simulink model "quadcopter_rl_env"  (R2024b)
settings: Solver=ode4  StartTime=0.0  StopTime=T_episode  FixedStep=Ts_inner  RelTol=1e-3
undefined symbols (not defined in the file): alpha, Kd_phi, Kd_psi, Kd_theta, Kd_x, Kd_y, Kd_z, Ki_phi, Ki_psi, Ki_theta, Ki_x, Ki_y, Ki_z, Kp_phi, Kp_psi, Kp_theta, Kp_x, Kp_y, Kp_z, psi_d, wind_force_N, wind_onset_time, x_d, y_d, z_d
libraries: slpidlib x6, rllib x1
settings Model: Creator=hridd  LastModifiedBy=hridd

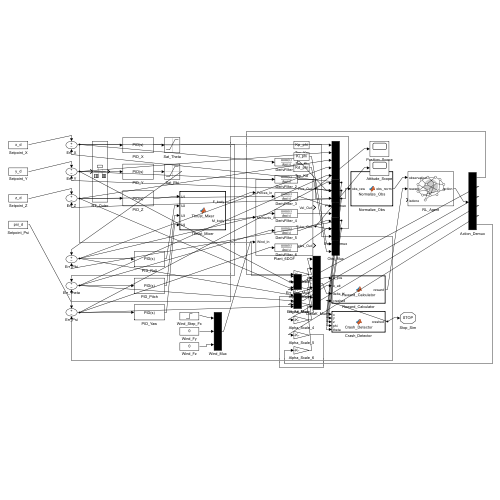
[thumbnail: Simulink's stored preview of the top-level diagram]
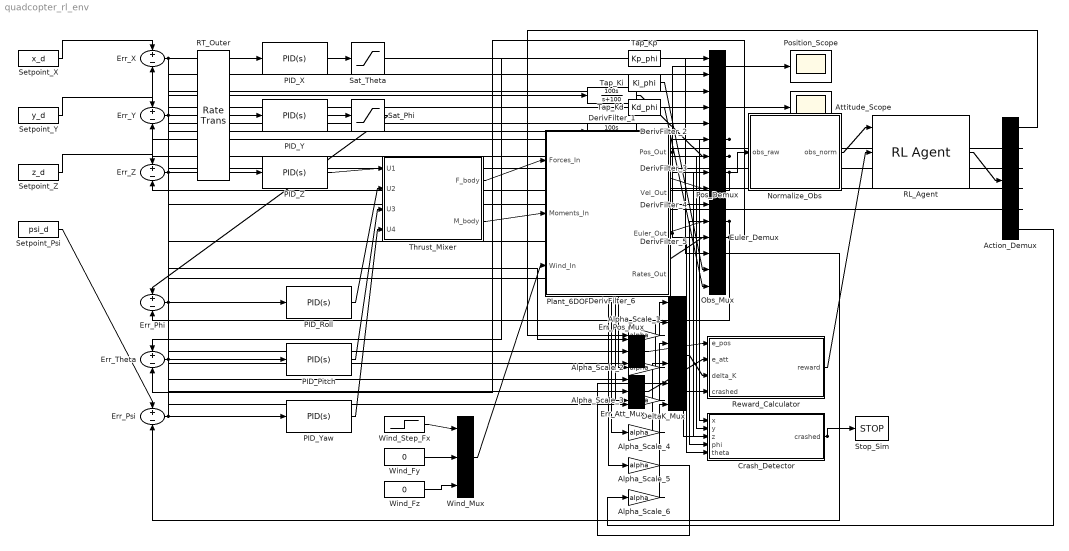
== system quadcopter_rl_env ==
  Action_Demux : Demux  Outputs=6
  Alpha_Scale_{1..6} (6 alike) : Gain  Gain=alpha
  Attitude_Scope : Scope
  Crash_Detector : MATLAB Function  TreatAsAtomicUnit=on
  DeltaK_Mux : Mux  Inputs=6
  DerivFilter_{1..6} (6 alike) : TransferFcn  Numerator=[100 0]  Denominator=[1 100]
  Err_Att_Mux : Mux  Inputs=3
  Err_Phi : Sum  Inputs=+-
  Err_Pos_Mux : Mux  Inputs=3
  Err_Psi : Sum  Inputs=+-
  Err_Theta : Sum  Inputs=+-
  Err_X : Sum  Inputs=+-
  Err_Y : Sum  Inputs=+-
  Err_Z : Sum  Inputs=+-
  Euler_Demux : Demux  Outputs=3
  Normalize_Obs : MATLAB Function  TreatAsAtomicUnit=on
  Obs_Mux : Mux  Inputs=15
  PID_Pitch : slpidlib/PID Controller  Controller=PID  Form=Parallel  TimeDomain=Continuous-time  UseExternalTs=off  SampleTime=-1  IntegratorMethod=Forward Euler  FilterMethod=Forward Euler  ControllerParametersSource=internal  P=Kp_theta  I=Ki_theta  UseKiTs=off  D=Kd_theta  UseExternalDerivativeSource=off  N=100  UseFilter=on  TunerSelectOption=Transfer Function Based (PID Tuner App)  InitialConditionSource=internal  InitialConditionForIntegrator=0  InitialConditionForFilter=0  DifferentiatorICPrevScaledInput=0  ExternalReset=none  TrackingMode=off  Kt=1  LimitOutput=off  SatLimitsSource=internal  UpperSaturationLimit=inf  LowerSaturationLimit=-inf  LinearizeAsGain=on  AntiWindupMode=none  Kb=1  LimitIntegrator=off  UpperIntegratorSaturationLimit=inf  LowerIntegratorSaturationLimit=-inf  POutMin=[]  POutMax=[]  IOutMin=[]  IOutMax=[]  DOutMin=[]  DOutMax=[]  NOutMin=[]  NOutMax=[]  SumOutMin=[]  SumOutMax=[]  SaturationOutMin=[]  SaturationOutMax=[]  PParamMin=[]  PParamMax=[]  IParamMin=[]  IParamMax=[]  DParamMin=[]  DParamMax=[]  NParamMin=[]  NParamMax=[]  KbParamMin=[]  KbParamMax=[]  KtParamMin=[]  KtParamMax=[]  KbOutMin=[]  KbOutMax=[]  KtOutMin=[]  KtOutMax=[]  IntegratorOutMin=[]  IntegratorOutMax=[]  FilterOutMin=[]  FilterOutMax=[]  SumI1OutMin=[]  SumI1OutMax=[]  SumI2OutMin=[]  SumI2OutMax=[]  SumI3OutMin=[]  SumI3OutMax=[]  SumI4OutMin=[]  SumI4OutMax=[]  SumDOutMin=[]  SumDOutMax=[]  DifferentiatorOutMin=[]  DifferentiatorOutMax=[]  FilterDiffOutCoefMin=[]  FilterDiffOutCoefMax=[]  ReciprocalOutMin=[]  ReciprocalOutMax=[]  SumDenOutMin=[]  SumDenOutMax=[]  SumNumOutMin=[]  SumNumOutMax=[]  DivideOutMin=[]  DivideOutMax=[]  UdiffTsProdOutMin=[]  UdiffTsProdOutMax=[]  NTsProdOutMin=[]  NTsProdOutMax=[]  UintegralTsProdOutMin=[]  UintegralTsProdOutMax=[]  UngainTsProdOutMin=[]  UngainTsProdOutMax=[]  ClampingZeroOutDataTypeStr=Inherit: Inherit via back propagation  ClampingZeroOutMin=[]  ClampingZeroOutMax=[]  FilterDenConstantOutDataTypeStr=Inherit: Inherit via back propagation  FilterDenConstantOutMin=[]  FilterDenConstantOutMax=[]  PCopyOutDataTypeStr=Inherit: Inherit via back propagation  PCopyOutMin=[]  PCopyOutMax=[]  NCopyOutDataTypeStr=Inherit: Inherit via back propagation  NCopyOutMin=[]  NCopyOutMax=[]  IntegratorContinuousStateAttributes=''  IntegratorStateMustResolveToSignalObject=off  IntegratorRTWStateStorageClass=Auto  FilterContinuousStateAttributes=''  FilterStateMustResolveToSignalObject=off  FilterRTWStateStorageClass=Auto  ParallelPVariant=InternalParameters  IdealPVariant=Disabled  IVariant=InternalParameters  DVariant=InternalParameters  IntegratorVariant=Continuous  SatVariant=Disabled  AWVariant=Passthrough  PCopyVariant=Disabled  TRVariant=Disabled  FdbkBlocksVariant=Forward  IdealPFdbkVariant=Disabled  SatFdbkVariant=Disabled  DerivativeFilterVariant=ContFilter  NVariant=InternalParameters  NCopyVariant=Disabled  FilterICVariant=InternalICsFilter  IntegratorICVariant=InternalICs  ExternalResetVariant=Disabled  TRSumVariant=Passthrough  SumFdbkVariant=Disabled  SumVariant=Sum_PID  TsampFilterVariant=InternalTs  TsampNgainVariant=Passthrough  TsampIntegralVariant=Disabled_SignalSpec  ExternalSaturationOutDataTypeStr=Inherit: Same as second input  DerivativeSourceVariant=ErrorSignal  PreIntVariant=InternalPreInt
  PID_Roll : slpidlib/PID Controller  Controller=PID  Form=Parallel  TimeDomain=Continuous-time  UseExternalTs=off  SampleTime=-1  IntegratorMethod=Forward Euler  FilterMethod=Forward Euler  ControllerParametersSource=internal  P=Kp_phi  I=Ki_phi  UseKiTs=off  D=Kd_phi  UseExternalDerivativeSource=off  N=100  UseFilter=on  TunerSelectOption=Transfer Function Based (PID Tuner App)  InitialConditionSource=internal  InitialConditionForIntegrator=0  InitialConditionForFilter=0  DifferentiatorICPrevScaledInput=0  ExternalReset=none  TrackingMode=off  Kt=1  LimitOutput=off  SatLimitsSource=internal  UpperSaturationLimit=inf  LowerSaturationLimit=-inf  LinearizeAsGain=on  AntiWindupMode=none  Kb=1  LimitIntegrator=off  UpperIntegratorSaturationLimit=inf  LowerIntegratorSaturationLimit=-inf  POutMin=[]  POutMax=[]  IOutMin=[]  IOutMax=[]  DOutMin=[]  DOutMax=[]  NOutMin=[]  NOutMax=[]  SumOutMin=[]  SumOutMax=[]  SaturationOutMin=[]  SaturationOutMax=[]  PParamMin=[]  PParamMax=[]  IParamMin=[]  IParamMax=[]  DParamMin=[]  DParamMax=[]  NParamMin=[]  NParamMax=[]  KbParamMin=[]  KbParamMax=[]  KtParamMin=[]  KtParamMax=[]  KbOutMin=[]  KbOutMax=[]  KtOutMin=[]  KtOutMax=[]  IntegratorOutMin=[]  IntegratorOutMax=[]  FilterOutMin=[]  FilterOutMax=[]  SumI1OutMin=[]  SumI1OutMax=[]  SumI2OutMin=[]  SumI2OutMax=[]  SumI3OutMin=[]  SumI3OutMax=[]  SumI4OutMin=[]  SumI4OutMax=[]  SumDOutMin=[]  SumDOutMax=[]  DifferentiatorOutMin=[]  DifferentiatorOutMax=[]  FilterDiffOutCoefMin=[]  FilterDiffOutCoefMax=[]  ReciprocalOutMin=[]  ReciprocalOutMax=[]  SumDenOutMin=[]  SumDenOutMax=[]  SumNumOutMin=[]  SumNumOutMax=[]  DivideOutMin=[]  DivideOutMax=[]  UdiffTsProdOutMin=[]  UdiffTsProdOutMax=[]  NTsProdOutMin=[]  NTsProdOutMax=[]  UintegralTsProdOutMin=[]  UintegralTsProdOutMax=[]  UngainTsProdOutMin=[]  UngainTsProdOutMax=[]  ClampingZeroOutDataTypeStr=Inherit: Inherit via back propagation  ClampingZeroOutMin=[]  ClampingZeroOutMax=[]  FilterDenConstantOutDataTypeStr=Inherit: Inherit via back propagation  FilterDenConstantOutMin=[]  FilterDenConstantOutMax=[]  PCopyOutDataTypeStr=Inherit: Inherit via back propagation  PCopyOutMin=[]  PCopyOutMax=[]  NCopyOutDataTypeStr=Inherit: Inherit via back propagation  NCopyOutMin=[]  NCopyOutMax=[]  IntegratorContinuousStateAttributes=''  IntegratorStateMustResolveToSignalObject=off  IntegratorRTWStateStorageClass=Auto  FilterContinuousStateAttributes=''  FilterStateMustResolveToSignalObject=off  FilterRTWStateStorageClass=Auto  ParallelPVariant=InternalParameters  IdealPVariant=Disabled  IVariant=InternalParameters  DVariant=InternalParameters  IntegratorVariant=Continuous  SatVariant=Disabled  AWVariant=Passthrough  PCopyVariant=Disabled  TRVariant=Disabled  FdbkBlocksVariant=Forward  IdealPFdbkVariant=Disabled  SatFdbkVariant=Disabled  DerivativeFilterVariant=ContFilter  NVariant=InternalParameters  NCopyVariant=Disabled  FilterICVariant=InternalICsFilter  IntegratorICVariant=InternalICs  ExternalResetVariant=Disabled  TRSumVariant=Passthrough  SumFdbkVariant=Disabled  SumVariant=Sum_PID  TsampFilterVariant=InternalTs  TsampNgainVariant=Passthrough  TsampIntegralVariant=Disabled_SignalSpec  ExternalSaturationOutDataTypeStr=Inherit: Same as second input  DerivativeSourceVariant=ErrorSignal  PreIntVariant=InternalPreInt
  PID_X : slpidlib/PID Controller  Controller=PID  Form=Parallel  TimeDomain=Continuous-time  UseExternalTs=off  SampleTime=-1  IntegratorMethod=Forward Euler  FilterMethod=Forward Euler  ControllerParametersSource=internal  P=Kp_x  I=Ki_x  UseKiTs=off  D=Kd_x  UseExternalDerivativeSource=off  N=100  UseFilter=on  TunerSelectOption=Transfer Function Based (PID Tuner App)  InitialConditionSource=internal  InitialConditionForIntegrator=0  InitialConditionForFilter=0  DifferentiatorICPrevScaledInput=0  ExternalReset=none  TrackingMode=off  Kt=1  LimitOutput=off  SatLimitsSource=internal  UpperSaturationLimit=inf  LowerSaturationLimit=-inf  LinearizeAsGain=on  AntiWindupMode=none  Kb=1  LimitIntegrator=off  UpperIntegratorSaturationLimit=inf  LowerIntegratorSaturationLimit=-inf  POutMin=[]  POutMax=[]  IOutMin=[]  IOutMax=[]  DOutMin=[]  DOutMax=[]  NOutMin=[]  NOutMax=[]  SumOutMin=[]  SumOutMax=[]  SaturationOutMin=[]  SaturationOutMax=[]  PParamMin=[]  PParamMax=[]  IParamMin=[]  IParamMax=[]  DParamMin=[]  DParamMax=[]  NParamMin=[]  NParamMax=[]  KbParamMin=[]  KbParamMax=[]  KtParamMin=[]  KtParamMax=[]  KbOutMin=[]  KbOutMax=[]  KtOutMin=[]  KtOutMax=[]  IntegratorOutMin=[]  IntegratorOutMax=[]  FilterOutMin=[]  FilterOutMax=[]  SumI1OutMin=[]  SumI1OutMax=[]  SumI2OutMin=[]  SumI2OutMax=[]  SumI3OutMin=[]  SumI3OutMax=[]  SumI4OutMin=[]  SumI4OutMax=[]  SumDOutMin=[]  SumDOutMax=[]  DifferentiatorOutMin=[]  DifferentiatorOutMax=[]  FilterDiffOutCoefMin=[]  FilterDiffOutCoefMax=[]  ReciprocalOutMin=[]  ReciprocalOutMax=[]  SumDenOutMin=[]  SumDenOutMax=[]  SumNumOutMin=[]  SumNumOutMax=[]  DivideOutMin=[]  DivideOutMax=[]  UdiffTsProdOutMin=[]  UdiffTsProdOutMax=[]  NTsProdOutMin=[]  NTsProdOutMax=[]  UintegralTsProdOutMin=[]  UintegralTsProdOutMax=[]  UngainTsProdOutMin=[]  UngainTsProdOutMax=[]  ClampingZeroOutDataTypeStr=Inherit: Inherit via back propagation  ClampingZeroOutMin=[]  ClampingZeroOutMax=[]  FilterDenConstantOutDataTypeStr=Inherit: Inherit via back propagation  FilterDenConstantOutMin=[]  FilterDenConstantOutMax=[]  PCopyOutDataTypeStr=Inherit: Inherit via back propagation  PCopyOutMin=[]  PCopyOutMax=[]  NCopyOutDataTypeStr=Inherit: Inherit via back propagation  NCopyOutMin=[]  NCopyOutMax=[]  IntegratorContinuousStateAttributes=''  IntegratorStateMustResolveToSignalObject=off  IntegratorRTWStateStorageClass=Auto  FilterContinuousStateAttributes=''  FilterStateMustResolveToSignalObject=off  FilterRTWStateStorageClass=Auto  ParallelPVariant=InternalParameters  IdealPVariant=Disabled  IVariant=InternalParameters  DVariant=InternalParameters  IntegratorVariant=Continuous  SatVariant=Disabled  AWVariant=Passthrough  PCopyVariant=Disabled  TRVariant=Disabled  FdbkBlocksVariant=Forward  IdealPFdbkVariant=Disabled  SatFdbkVariant=Disabled  DerivativeFilterVariant=ContFilter  NVariant=InternalParameters  NCopyVariant=Disabled  FilterICVariant=InternalICsFilter  IntegratorICVariant=InternalICs  ExternalResetVariant=Disabled  TRSumVariant=Passthrough  SumFdbkVariant=Disabled  SumVariant=Sum_PID  TsampFilterVariant=InternalTs  TsampNgainVariant=Passthrough  TsampIntegralVariant=Disabled_SignalSpec  ExternalSaturationOutDataTypeStr=Inherit: Same as second input  DerivativeSourceVariant=ErrorSignal  PreIntVariant=InternalPreInt
  PID_Y : slpidlib/PID Controller  Controller=PID  Form=Parallel  TimeDomain=Continuous-time  UseExternalTs=off  SampleTime=-1  IntegratorMethod=Forward Euler  FilterMethod=Forward Euler  ControllerParametersSource=internal  P=Kp_y  I=Ki_y  UseKiTs=off  D=Kd_y  UseExternalDerivativeSource=off  N=100  UseFilter=on  TunerSelectOption=Transfer Function Based (PID Tuner App)  InitialConditionSource=internal  InitialConditionForIntegrator=0  InitialConditionForFilter=0  DifferentiatorICPrevScaledInput=0  ExternalReset=none  TrackingMode=off  Kt=1  LimitOutput=off  SatLimitsSource=internal  UpperSaturationLimit=inf  LowerSaturationLimit=-inf  LinearizeAsGain=on  AntiWindupMode=none  Kb=1  LimitIntegrator=off  UpperIntegratorSaturationLimit=inf  LowerIntegratorSaturationLimit=-inf  POutMin=[]  POutMax=[]  IOutMin=[]  IOutMax=[]  DOutMin=[]  DOutMax=[]  NOutMin=[]  NOutMax=[]  SumOutMin=[]  SumOutMax=[]  SaturationOutMin=[]  SaturationOutMax=[]  PParamMin=[]  PParamMax=[]  IParamMin=[]  IParamMax=[]  DParamMin=[]  DParamMax=[]  NParamMin=[]  NParamMax=[]  KbParamMin=[]  KbParamMax=[]  KtParamMin=[]  KtParamMax=[]  KbOutMin=[]  KbOutMax=[]  KtOutMin=[]  KtOutMax=[]  IntegratorOutMin=[]  IntegratorOutMax=[]  FilterOutMin=[]  FilterOutMax=[]  SumI1OutMin=[]  SumI1OutMax=[]  SumI2OutMin=[]  SumI2OutMax=[]  SumI3OutMin=[]  SumI3OutMax=[]  SumI4OutMin=[]  SumI4OutMax=[]  SumDOutMin=[]  SumDOutMax=[]  DifferentiatorOutMin=[]  DifferentiatorOutMax=[]  FilterDiffOutCoefMin=[]  FilterDiffOutCoefMax=[]  ReciprocalOutMin=[]  ReciprocalOutMax=[]  SumDenOutMin=[]  SumDenOutMax=[]  SumNumOutMin=[]  SumNumOutMax=[]  DivideOutMin=[]  DivideOutMax=[]  UdiffTsProdOutMin=[]  UdiffTsProdOutMax=[]  NTsProdOutMin=[]  NTsProdOutMax=[]  UintegralTsProdOutMin=[]  UintegralTsProdOutMax=[]  UngainTsProdOutMin=[]  UngainTsProdOutMax=[]  ClampingZeroOutDataTypeStr=Inherit: Inherit via back propagation  ClampingZeroOutMin=[]  ClampingZeroOutMax=[]  FilterDenConstantOutDataTypeStr=Inherit: Inherit via back propagation  FilterDenConstantOutMin=[]  FilterDenConstantOutMax=[]  PCopyOutDataTypeStr=Inherit: Inherit via back propagation  PCopyOutMin=[]  PCopyOutMax=[]  NCopyOutDataTypeStr=Inherit: Inherit via back propagation  NCopyOutMin=[]  NCopyOutMax=[]  IntegratorContinuousStateAttributes=''  IntegratorStateMustResolveToSignalObject=off  IntegratorRTWStateStorageClass=Auto  FilterContinuousStateAttributes=''  FilterStateMustResolveToSignalObject=off  FilterRTWStateStorageClass=Auto  ParallelPVariant=InternalParameters  IdealPVariant=Disabled  IVariant=InternalParameters  DVariant=InternalParameters  IntegratorVariant=Continuous  SatVariant=Disabled  AWVariant=Passthrough  PCopyVariant=Disabled  TRVariant=Disabled  FdbkBlocksVariant=Forward  IdealPFdbkVariant=Disabled  SatFdbkVariant=Disabled  DerivativeFilterVariant=ContFilter  NVariant=InternalParameters  NCopyVariant=Disabled  FilterICVariant=InternalICsFilter  IntegratorICVariant=InternalICs  ExternalResetVariant=Disabled  TRSumVariant=Passthrough  SumFdbkVariant=Disabled  SumVariant=Sum_PID  TsampFilterVariant=InternalTs  TsampNgainVariant=Passthrough  TsampIntegralVariant=Disabled_SignalSpec  ExternalSaturationOutDataTypeStr=Inherit: Same as second input  DerivativeSourceVariant=ErrorSignal  PreIntVariant=InternalPreInt
  PID_Yaw : slpidlib/PID Controller  Controller=PID  Form=Parallel  TimeDomain=Continuous-time  UseExternalTs=off  SampleTime=-1  IntegratorMethod=Forward Euler  FilterMethod=Forward Euler  ControllerParametersSource=internal  P=Kp_psi  I=Ki_psi  UseKiTs=off  D=Kd_psi  UseExternalDerivativeSource=off  N=100  UseFilter=on  TunerSelectOption=Transfer Function Based (PID Tuner App)  InitialConditionSource=internal  InitialConditionForIntegrator=0  InitialConditionForFilter=0  DifferentiatorICPrevScaledInput=0  ExternalReset=none  TrackingMode=off  Kt=1  LimitOutput=off  SatLimitsSource=internal  UpperSaturationLimit=inf  LowerSaturationLimit=-inf  LinearizeAsGain=on  AntiWindupMode=none  Kb=1  LimitIntegrator=off  UpperIntegratorSaturationLimit=inf  LowerIntegratorSaturationLimit=-inf  POutMin=[]  POutMax=[]  IOutMin=[]  IOutMax=[]  DOutMin=[]  DOutMax=[]  NOutMin=[]  NOutMax=[]  SumOutMin=[]  SumOutMax=[]  SaturationOutMin=[]  SaturationOutMax=[]  PParamMin=[]  PParamMax=[]  IParamMin=[]  IParamMax=[]  DParamMin=[]  DParamMax=[]  NParamMin=[]  NParamMax=[]  KbParamMin=[]  KbParamMax=[]  KtParamMin=[]  KtParamMax=[]  KbOutMin=[]  KbOutMax=[]  KtOutMin=[]  KtOutMax=[]  IntegratorOutMin=[]  IntegratorOutMax=[]  FilterOutMin=[]  FilterOutMax=[]  SumI1OutMin=[]  SumI1OutMax=[]  SumI2OutMin=[]  SumI2OutMax=[]  SumI3OutMin=[]  SumI3OutMax=[]  SumI4OutMin=[]  SumI4OutMax=[]  SumDOutMin=[]  SumDOutMax=[]  DifferentiatorOutMin=[]  DifferentiatorOutMax=[]  FilterDiffOutCoefMin=[]  FilterDiffOutCoefMax=[]  ReciprocalOutMin=[]  ReciprocalOutMax=[]  SumDenOutMin=[]  SumDenOutMax=[]  SumNumOutMin=[]  SumNumOutMax=[]  DivideOutMin=[]  DivideOutMax=[]  UdiffTsProdOutMin=[]  UdiffTsProdOutMax=[]  NTsProdOutMin=[]  NTsProdOutMax=[]  UintegralTsProdOutMin=[]  UintegralTsProdOutMax=[]  UngainTsProdOutMin=[]  UngainTsProdOutMax=[]  ClampingZeroOutDataTypeStr=Inherit: Inherit via back propagation  ClampingZeroOutMin=[]  ClampingZeroOutMax=[]  FilterDenConstantOutDataTypeStr=Inherit: Inherit via back propagation  FilterDenConstantOutMin=[]  FilterDenConstantOutMax=[]  PCopyOutDataTypeStr=Inherit: Inherit via back propagation  PCopyOutMin=[]  PCopyOutMax=[]  NCopyOutDataTypeStr=Inherit: Inherit via back propagation  NCopyOutMin=[]  NCopyOutMax=[]  IntegratorContinuousStateAttributes=''  IntegratorStateMustResolveToSignalObject=off  IntegratorRTWStateStorageClass=Auto  FilterContinuousStateAttributes=''  FilterStateMustResolveToSignalObject=off  FilterRTWStateStorageClass=Auto  ParallelPVariant=InternalParameters  IdealPVariant=Disabled  IVariant=InternalParameters  DVariant=InternalParameters  IntegratorVariant=Continuous  SatVariant=Disabled  AWVariant=Passthrough  PCopyVariant=Disabled  TRVariant=Disabled  FdbkBlocksVariant=Forward  IdealPFdbkVariant=Disabled  SatFdbkVariant=Disabled  DerivativeFilterVariant=ContFilter  NVariant=InternalParameters  NCopyVariant=Disabled  FilterICVariant=InternalICsFilter  IntegratorICVariant=InternalICs  ExternalResetVariant=Disabled  TRSumVariant=Passthrough  SumFdbkVariant=Disabled  SumVariant=Sum_PID  TsampFilterVariant=InternalTs  TsampNgainVariant=Passthrough  TsampIntegralVariant=Disabled_SignalSpec  ExternalSaturationOutDataTypeStr=Inherit: Same as second input  DerivativeSourceVariant=ErrorSignal  PreIntVariant=InternalPreInt
  PID_Z : slpidlib/PID Controller  Controller=PID  Form=Parallel  TimeDomain=Continuous-time  UseExternalTs=off  SampleTime=-1  IntegratorMethod=Forward Euler  FilterMethod=Forward Euler  ControllerParametersSource=internal  P=Kp_z  I=Ki_z  UseKiTs=off  D=Kd_z  UseExternalDerivativeSource=off  N=100  UseFilter=on  TunerSelectOption=Transfer Function Based (PID Tuner App)  InitialConditionSource=internal  InitialConditionForIntegrator=0  InitialConditionForFilter=0  DifferentiatorICPrevScaledInput=0  ExternalReset=none  TrackingMode=off  Kt=1  LimitOutput=off  SatLimitsSource=internal  UpperSaturationLimit=inf  LowerSaturationLimit=-inf  LinearizeAsGain=on  AntiWindupMode=none  Kb=1  LimitIntegrator=off  UpperIntegratorSaturationLimit=inf  LowerIntegratorSaturationLimit=-inf  POutMin=[]  POutMax=[]  IOutMin=[]  IOutMax=[]  DOutMin=[]  DOutMax=[]  NOutMin=[]  NOutMax=[]  SumOutMin=[]  SumOutMax=[]  SaturationOutMin=[]  SaturationOutMax=[]  PParamMin=[]  PParamMax=[]  IParamMin=[]  IParamMax=[]  DParamMin=[]  DParamMax=[]  NParamMin=[]  NParamMax=[]  KbParamMin=[]  KbParamMax=[]  KtParamMin=[]  KtParamMax=[]  KbOutMin=[]  KbOutMax=[]  KtOutMin=[]  KtOutMax=[]  IntegratorOutMin=[]  IntegratorOutMax=[]  FilterOutMin=[]  FilterOutMax=[]  SumI1OutMin=[]  SumI1OutMax=[]  SumI2OutMin=[]  SumI2OutMax=[]  SumI3OutMin=[]  SumI3OutMax=[]  SumI4OutMin=[]  SumI4OutMax=[]  SumDOutMin=[]  SumDOutMax=[]  DifferentiatorOutMin=[]  DifferentiatorOutMax=[]  FilterDiffOutCoefMin=[]  FilterDiffOutCoefMax=[]  ReciprocalOutMin=[]  ReciprocalOutMax=[]  SumDenOutMin=[]  SumDenOutMax=[]  SumNumOutMin=[]  SumNumOutMax=[]  DivideOutMin=[]  DivideOutMax=[]  UdiffTsProdOutMin=[]  UdiffTsProdOutMax=[]  NTsProdOutMin=[]  NTsProdOutMax=[]  UintegralTsProdOutMin=[]  UintegralTsProdOutMax=[]  UngainTsProdOutMin=[]  UngainTsProdOutMax=[]  ClampingZeroOutDataTypeStr=Inherit: Inherit via back propagation  ClampingZeroOutMin=[]  ClampingZeroOutMax=[]  FilterDenConstantOutDataTypeStr=Inherit: Inherit via back propagation  FilterDenConstantOutMin=[]  FilterDenConstantOutMax=[]  PCopyOutDataTypeStr=Inherit: Inherit via back propagation  PCopyOutMin=[]  PCopyOutMax=[]  NCopyOutDataTypeStr=Inherit: Inherit via back propagation  NCopyOutMin=[]  NCopyOutMax=[]  IntegratorContinuousStateAttributes=''  IntegratorStateMustResolveToSignalObject=off  IntegratorRTWStateStorageClass=Auto  FilterContinuousStateAttributes=''  FilterStateMustResolveToSignalObject=off  FilterRTWStateStorageClass=Auto  ParallelPVariant=InternalParameters  IdealPVariant=Disabled  IVariant=InternalParameters  DVariant=InternalParameters  IntegratorVariant=Continuous  SatVariant=Disabled  AWVariant=Passthrough  PCopyVariant=Disabled  TRVariant=Disabled  FdbkBlocksVariant=Forward  IdealPFdbkVariant=Disabled  SatFdbkVariant=Disabled  DerivativeFilterVariant=ContFilter  NVariant=InternalParameters  NCopyVariant=Disabled  FilterICVariant=InternalICsFilter  IntegratorICVariant=InternalICs  ExternalResetVariant=Disabled  TRSumVariant=Passthrough  SumFdbkVariant=Disabled  SumVariant=Sum_PID  TsampFilterVariant=InternalTs  TsampNgainVariant=Passthrough  TsampIntegralVariant=Disabled_SignalSpec  ExternalSaturationOutDataTypeStr=Inherit: Same as second input  DerivativeSourceVariant=ErrorSignal  PreIntVariant=InternalPreInt
  Plant_6DOF : Subsystem
  Pos_Demux : Demux  Outputs=3
  Position_Scope : Scope
  RL_Agent : rllib/RL Agent  Agent=agentObj  ExternalActionAsInput=off  ProvideLastAction=off  ProvideCumRwd=off  TreatAsDirectFeedthrough=on  UseStrictObservationDataTypes=off
  RT_Outer : RateTransition  OutPortSampleTime=Ts_outer
  Reward_Calculator : MATLAB Function  TreatAsAtomicUnit=on
  Sat_Phi : Saturate  UpperLimit=0.3  LowerLimit=-0.3
  Sat_Theta : Saturate  UpperLimit=0.3  LowerLimit=-0.3
  Setpoint_Psi : Constant  Value=psi_d
  Setpoint_X : Constant  Value=x_d
  Setpoint_Y : Constant  Value=y_d
  Setpoint_Z : Constant  Value=z_d
  Stop_Sim : Stop
  Tap_Kd : Constant  Value=Kd_phi
  Tap_Ki : Constant  Value=Ki_phi
  Tap_Kp : Constant  Value=Kp_phi
  Thrust_Mixer : MATLAB Function  TreatAsAtomicUnit=on
  Wind_Fy : Constant  Value=0
  Wind_Fz : Constant  Value=0
  Wind_Mux : Mux  Inputs=3
  Wind_Step_Fx : Step  Time=wind_onset_time  After=wind_force_N  SampleTime=0
  wires:
  Setpoint_X/1 -> Err_X/1
  Setpoint_Y/1 -> Err_Y/1
  Setpoint_Z/1 -> Err_Z/1
  Setpoint_Psi/1 -> Err_Psi/1
  Err_X/1 -> PID_X/1, Obs_Mux/1, DerivFilter_1/1, Err_Pos_Mux/1
  Err_Y/1 -> PID_Y/1, Obs_Mux/2, DerivFilter_2/1, Err_Pos_Mux/2
  Err_Z/1 -> PID_Z/1, Obs_Mux/3, DerivFilter_3/1, Err_Pos_Mux/3
  PID_X/1 -> Sat_Theta/1
  PID_Y/1 -> Sat_Phi/1
  Sat_Phi/1 -> Err_Phi/1
  Sat_Theta/1 -> Err_Theta/1
  Err_Phi/1 -> PID_Roll/1, Obs_Mux/4, DerivFilter_4/1, Err_Att_Mux/1
  Err_Theta/1 -> PID_Pitch/1, Obs_Mux/5, DerivFilter_5/1, Err_Att_Mux/2
  Err_Psi/1 -> PID_Yaw/1, Obs_Mux/6, DerivFilter_6/1, Err_Att_Mux/3
  PID_Z/1 -> Thrust_Mixer/1(U1)
  PID_Roll/1 -> Thrust_Mixer/2(U2)
  PID_Pitch/1 -> Thrust_Mixer/3(U3)
  PID_Yaw/1 -> Thrust_Mixer/4(U4)
  Thrust_Mixer/1(F_body) -> Plant_6DOF/1(Forces_In)
  Thrust_Mixer/2(M_body) -> Plant_6DOF/2(Moments_In)
  Wind_Step_Fx/1 -> Wind_Mux/1
  Wind_Fy/1 -> Wind_Mux/2
  Wind_Fz/1 -> Wind_Mux/3
  Wind_Mux/1 -> Plant_6DOF/3(Wind_In)
  Plant_6DOF/1(Pos_Out) -> Pos_Demux/1, Position_Scope/1
  Pos_Demux/1 -> Err_X/2, Crash_Detector/1(x)
  Pos_Demux/2 -> Err_Y/2, Crash_Detector/2(y)
  Pos_Demux/3 -> Err_Z/2, Crash_Detector/3(z)
  Plant_6DOF/3(Euler_Out) -> Euler_Demux/1, Attitude_Scope/1
  Euler_Demux/1 -> Err_Phi/2, Crash_Detector/4(phi)
  Euler_Demux/2 -> Err_Theta/2, Crash_Detector/5(theta)
  Euler_Demux/3 -> Err_Psi/2
  DerivFilter_1/1 -> Obs_Mux/7
  DerivFilter_2/1 -> Obs_Mux/8
  DerivFilter_3/1 -> Obs_Mux/9
  DerivFilter_4/1 -> Obs_Mux/10
  DerivFilter_5/1 -> Obs_Mux/11
  DerivFilter_6/1 -> Obs_Mux/12
  Tap_Kp/1 -> Obs_Mux/13
  Tap_Ki/1 -> Obs_Mux/14
  Tap_Kd/1 -> Obs_Mux/15
  Obs_Mux/1 -> Normalize_Obs/1(obs_raw)
  Normalize_Obs/1(obs_norm) -> RL_Agent/1
  Reward_Calculator/1(reward) -> RL_Agent/2
  RL_Agent/1 -> Action_Demux/1
  Action_Demux/1 -> Alpha_Scale_1/1
  Action_Demux/2 -> Alpha_Scale_2/1
  Action_Demux/3 -> Alpha_Scale_3/1
  Action_Demux/4 -> Alpha_Scale_4/1
  Action_Demux/5 -> Alpha_Scale_5/1
  Action_Demux/6 -> Alpha_Scale_6/1
  Alpha_Scale_1/1 -> DeltaK_Mux/1
  Alpha_Scale_2/1 -> DeltaK_Mux/2
  Alpha_Scale_3/1 -> DeltaK_Mux/3
  Alpha_Scale_4/1 -> DeltaK_Mux/4
  Alpha_Scale_5/1 -> DeltaK_Mux/5
  Alpha_Scale_6/1 -> DeltaK_Mux/6
  Err_Pos_Mux/1 -> Reward_Calculator/1(e_pos)
  Err_Att_Mux/1 -> Reward_Calculator/2(e_att)
  DeltaK_Mux/1 -> Reward_Calculator/3(delta_K)
  Crash_Detector/1(crashed) -> Reward_Calculator/4(crashed), Stop_Sim/1

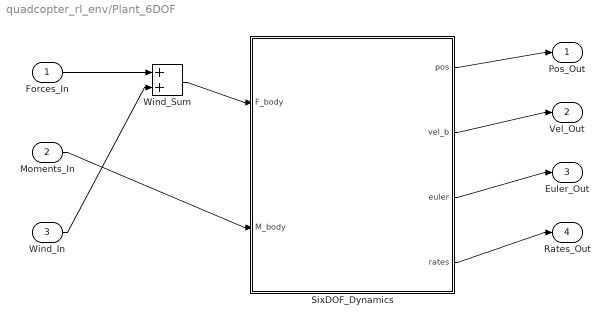
== system quadcopter_rl_env/Plant_6DOF ==
  Forces_In : Inport
  Moments_In : Inport  Port=2
  Wind_In : Inport  Port=3
  SixDOF_Dynamics : MATLAB Function  TreatAsAtomicUnit=on
  Wind_Sum : Sum
  Pos_Out : Outport
  Vel_Out : Outport  Port=2
  Euler_Out : Outport  Port=3
  Rates_Out : Outport  Port=4
  wires:
  Forces_In/1 -> Wind_Sum/1
  Wind_In/1 -> Wind_Sum/2
  Wind_Sum/1 -> SixDOF_Dynamics/1(F_body)
  Moments_In/1 -> SixDOF_Dynamics/2(M_body)
  SixDOF_Dynamics/1(pos) -> Pos_Out/1
  SixDOF_Dynamics/2(vel_b) -> Vel_Out/1
  SixDOF_Dynamics/3(euler) -> Euler_Out/1
  SixDOF_Dynamics/4(rates) -> Rates_Out/1

== matlab function quadcopter_rl_env/Thrust_Mixer ==
  data: U1 input; F_body output; U2 input; U3 input; U4 input; M_body output
function [F_body, M_body] = Thrust_Mixer(U1, U2, U3, U4)
%#codegen
F_body = [0; 0; -U1];
M_body = [U2; U3; U4];

== matlab function quadcopter_rl_env/Plant_6DOF/SixDOF_Dynamics ==
  data: F_body input; pos output; M_body input; vel_b output; euler output; rates output
function [pos, vel_b, euler, rates] = SixDOF_Dynamics(F_body, M_body)
%#codegen
F_body=F_body(:); M_body=M_body(:);
persistent x_state
if isempty(x_state); x_state=zeros(12,1); x_state(3)=-1; end
m_p=0.468000; g_p=9.8100;
Ixx_p=4.856000e-03; Iyy_p=4.856000e-03; Izz_p=8.801000e-03;
Ax_p=0.0100; Ay_p=0.0100; Az_p=0.0200; Ts_p=0.002000;
u_s=x_state(4); v_s=x_state(5); w_s=x_state(6);
phi_s=x_state(7); theta_s=x_state(8); psi_s=x_state(9);
p_s=x_state(10); q_s=x_state(11); r_s=x_state(12);
cphi=cos(phi_s); sphi=sin(phi_s); cth=cos(theta_s); sth=sin(theta_s); cpsi=cos(psi_s); spsi=sin(psi_s);
R11=cth*cpsi; R12=sphi*sth*cpsi-cphi*spsi; R13=cphi*sth*cpsi+sphi*spsi;
R21=cth*spsi; R22=sphi*sth*spsi+cphi*cpsi; R23=cphi*sth*spsi-sphi*cpsi;
R31=-sth; R32=sphi*cth; R33=cphi*cth;
Fn=zeros(3,1);
Fn(1)=R11*F_body(1)+R12*F_body(2)+R13*F_body(3);
Fn(2)=R21*F_body(1)+R22*F_body(2)+R23*F_body(3);
Fn(3)=R31*F_body(1)+R32*F_body(2)+R33*F_body(3)+m_p*g_p;
db=[-Ax_p*u_s;-Ay_p*v_s;-Az_p*w_s];
Dn=zeros(3,1);
Dn(1)=R11*db(1)+R12*db(2)+R13*db(3);
Dn(2)=R21*db(1)+R22*db(2)+R23*db(3);
Dn(3)=R31*db(1)+R32*db(2)+R33*db(3);
an=zeros(3,1);
an(1)=(Fn(1)+Dn(1))/m_p; an(2)=(Fn(2)+Dn(2))/m_p; an(3)=(Fn(3)+Dn(3))/m_p;
ab=zeros(3,1);
ab(1)=R11*an(1)+R21*an(2)+R31*an(3);
ab(2)=R12*an(1)+R22*an(2)+R32*an(3);
ab(3)=R13*an(1)+R23*an(2)+R33*an(3);
Iw1=Ixx_p*p_s; Iw2=Iyy_p*q_s; Iw3=Izz_p*r_s;
alr=zeros(3,1);
alr(1)=(M_body(1)-(q_s*Iw3-r_s*Iw2))/Ixx_p;
alr(2)=(M_body(2)-(r_s*Iw1-p_s*Iw3))/Iyy_p;
alr(3)=(M_body(3)-(p_s*Iw2-q_s*Iw1))/Izz_p;
cth_s=cth; if abs(cth_s)<1e-6; cth_s=1e-6; end
ed=zeros(3,1);
ed(1)=p_s+(sphi*sth/cth_s)*q_s+(cphi*sth/cth_s)*r_s;
ed(2)=cphi*q_s-sphi*r_s;
ed(3)=(sphi/cth_s)*q_s+(cphi/cth_s)*r_s;
vn=zeros(3,1);
vn(1)=R11*u_s+R12*v_s+R13*w_s;
vn(2)=R21*u_s+R22*v_s+R23*w_s;
vn(3)=R31*u_s+R32*v_s+R33*w_s;
x_state(1)=x_state(1)+vn(1)*Ts_p;
x_state(2)=x_state(2)+vn(2)*Ts_p;
x_state(3)=x_state(3)+vn(3)*Ts_p;
x_state(4)=x_state(4)+ab(1)*Ts_p;
x_state(5)=x_state(5)+ab(2)*Ts_p;
x_state(6)=x_state(6)+ab(3)*Ts_p;
x_state(7)=x_state(7)+ed(1)*Ts_p;
x_state(8)=x_state(8)+ed(2)*Ts_p;
x_state(9)=x_state(9)+ed(3)*Ts_p;
x_state(10)=x_state(10)+alr(1)*Ts_p;
x_state(11)=x_state(11)+alr(2)*Ts_p;
x_state(12)=x_state(12)+alr(3)*Ts_p;
pos=x_state(1:3); vel_b=x_state(4:6); euler=x_state(7:9); rates=x_state(10:12);

== matlab function quadcopter_rl_env/Normalize_Obs ==
  data: obs_raw input; obs_norm output
function obs_norm = Normalize_Obs(obs_raw)
%#codegen
obs_raw=obs_raw(:); obs_norm=zeros(15,1);
obs_norm(1:3)=obs_raw(1:3)/3.0;
obs_norm(4:6)=obs_raw(4:6)/0.5;
obs_norm(7:9)=obs_raw(7:9)/5.0;
obs_norm(10:12)=obs_raw(10:12)/3.0;
obs_norm(13)=obs_raw(13)/10.0;
obs_norm(14)=obs_raw(14)/2.0;
obs_norm(15)=obs_raw(15)/5.0;
obs_norm=max(min(obs_norm,1),-1);

== matlab function quadcopter_rl_env/Reward_Calculator ==
  data: e_pos input; reward output; e_att input; delta_K input; crashed input
function reward = Reward_Calculator(e_pos, e_att, delta_K, crashed)
%#codegen
e_pos=e_pos(:); e_att=e_att(:); delta_K=delta_K(:);
pc=0; for i=1:3; pc=pc+e_pos(i)*e_pos(i); end
ac=0; for i=1:3; ac=ac+e_att(i)*e_att(i); end
gc=0; for i=1:numel(delta_K); gc=gc+delta_K(i)*delta_K(i); end
pc=1.0*pc; ac=0.5*ac; gc=0.1*gc;
bonus=0; if pc<0.05 && ac<0.02; bonus=0.3; end
cc=double(crashed>0.5)*100.0;
reward=-(pc+ac+gc)+bonus-cc;
reward=max(min(reward,10.0),-110.0);

== matlab function quadcopter_rl_env/Crash_Detector ==
  data: x input; crashed output; y input; z input; phi input; theta input
function crashed = Crash_Detector(x, y, z, phi, theta)
%#codegen
pd=sqrt(x*x+y*y+(z-1)*(z-1));
ad=sqrt(phi*phi+theta*theta);
crashed=double(pd>3.0 || ad>1.2);
